simulink model "Simulation"  (R2024a)
settings: Solver=FixedStepAuto  StartTime=0.0  StopTime=0.5  FixedStep=0.1  RelTol=1e-3  EnableMultiTasking=on
settings Model: Creator=hp  LastModifiedBy=Dell

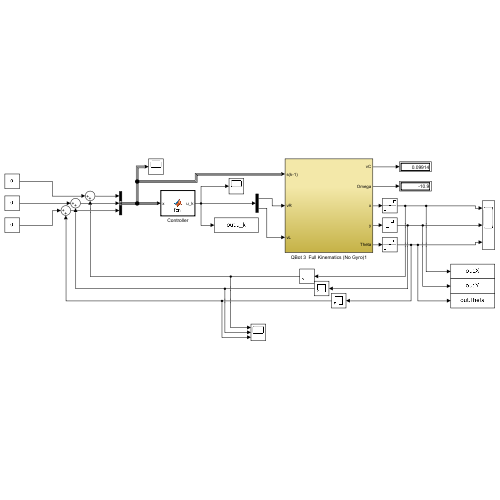
[thumbnail: Simulink's stored preview of the top-level diagram]
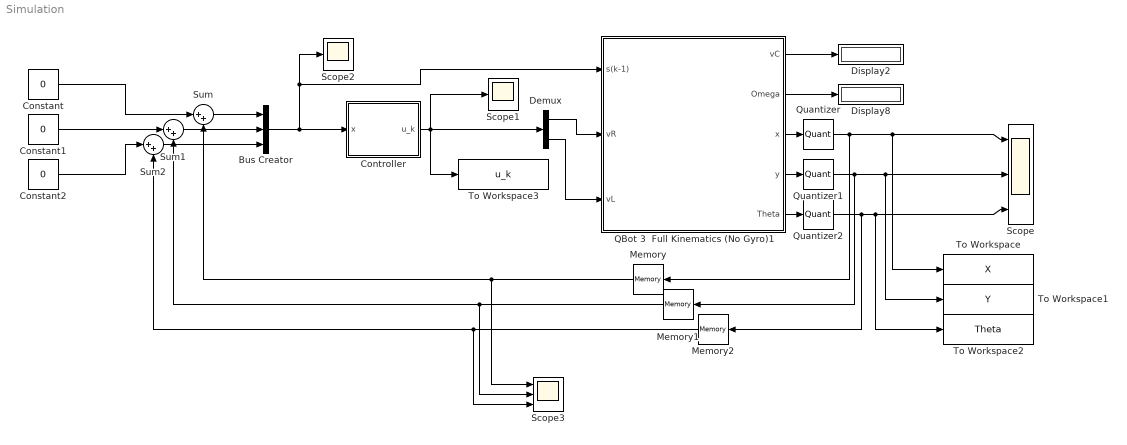
== system Simulation ==
  Bus Creator : BusCreator  Inputs=3
  Constant : Constant  Value=0
  Constant1 : Constant  Value=0
  Constant2 : Constant  Value=0
  Controller : MATLAB Function  TreatAsAtomicUnit=on
  Demux : Demux  Outputs=2
  Display2 : Display
  Display8 : Display
  Memory : Memory  InitialCondition=5
  Memory1 : Memory  InitialCondition=5
  Memory2 : Memory  InitialCondition=9
  QBot 3  Full Kinematics (No Gyro)1 : Subsystem
  Quantizer : Quantizer  QuantizationInterval=-1
  Quantizer1 : Quantizer  QuantizationInterval=-1
  Quantizer2 : Quantizer  QuantizationInterval=-1
  Scope : Scope  NumInputPorts=3
  Scope1 : Scope
  Scope2 : Scope
  Scope3 : Scope  NumInputPorts=3
  Sum : Sum  Inputs=|++
  Sum1 : Sum  Inputs=|++
  Sum2 : Sum  Inputs=|++
  To Workspace : ToWorkspace  VariableName=X  SaveFormat=Timeseries  SampleTime=-1
  To Workspace1 : ToWorkspace  VariableName=Y  SaveFormat=Timeseries  SampleTime=-1
  To Workspace2 : ToWorkspace  VariableName=Theta  SaveFormat=Timeseries  SampleTime=-1
  To Workspace3 : ToWorkspace  VariableName=u_k  SaveFormat=Timeseries  SampleTime=-1
  wires:
  QBot 3  Full Kinematics (No Gyro)1/2(Omega) -> Display8/1
  QBot 3  Full Kinematics (No Gyro)1/1(vC) -> Display2/1
  Demux/1 -> QBot 3  Full Kinematics (No Gyro)1/2(vR)
  Demux/2 -> QBot 3  Full Kinematics (No Gyro)1/3(vL)
  Bus Creator/1 -> QBot 3  Full Kinematics (No Gyro)1/1(s(k-1)), Scope2/1, Controller/1(x)
  Sum/1 -> Bus Creator/1
  Sum1/1 -> Bus Creator/2
  Sum2/1 -> Bus Creator/3
  Memory/1 -> Scope3/1, Sum/2
  Memory1/1 -> Scope3/2, Sum1/2
  Memory2/1 -> Scope3/3, Sum2/2
  Controller/1(u_k) -> Demux/1, Scope1/1, To Workspace3/1
  QBot 3  Full Kinematics (No Gyro)1/3(x) -> Quantizer/1
  QBot 3  Full Kinematics (No Gyro)1/4(y) -> Quantizer1/1
  QBot 3  Full Kinematics (No Gyro)1/5(Theta) -> Quantizer2/1
  Constant/1 -> Sum/1
  Constant1/1 -> Sum1/1
  Constant2/1 -> Sum2/1
  Quantizer/1 -> Memory/1, To Workspace/1, Scope/1
  Quantizer1/1 -> Memory1/1, To Workspace1/1, Scope/2
  Quantizer2/1 -> Memory2/1, To Workspace2/1, Scope/3

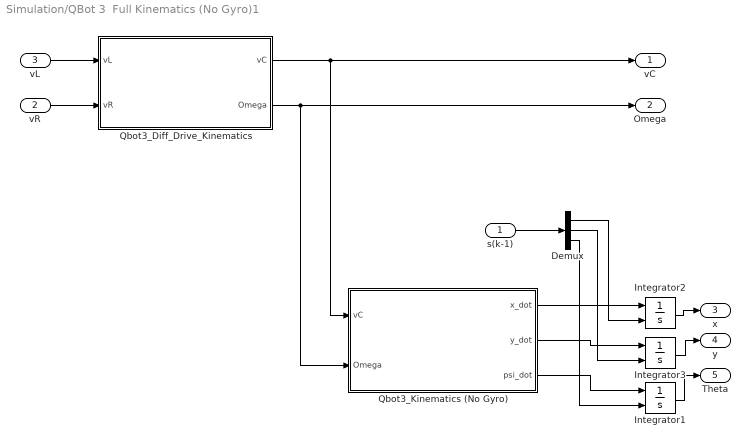
== system Simulation/QBot 3  Full Kinematics (No Gyro)1 ==
  s(k-1) : Inport
  vR : Inport  Port=2
  vL : Inport  Port=3
  Demux : Demux  Outputs=3
  Integrator1 : Integrator  InitialConditionSource=external  InitialCondition=9
  Integrator2 : Integrator  InitialConditionSource=external  InitialCondition=5
  Integrator3 : Integrator  InitialConditionSource=external  InitialCondition=5
  Qbot3_Diff_Drive_Kinematics : Subsystem
  Qbot3_Kinematics (No Gyro) : Subsystem
  vC : Outport
  Omega : Outport  Port=2
  x : Outport  Port=3
  y : Outport  Port=4
  Theta : Outport  Port=5
  wires:
  Qbot3_Kinematics (No Gyro)/2(y_dot) -> Integrator3/1
  Qbot3_Kinematics (No Gyro)/1(x_dot) -> Integrator2/1
  vL/1 -> Qbot3_Diff_Drive_Kinematics/1(vL)
  Qbot3_Diff_Drive_Kinematics/2(Omega) -> Omega/1, Qbot3_Kinematics (No Gyro)/2(Omega)
  Qbot3_Diff_Drive_Kinematics/1(vC) -> vC/1, Qbot3_Kinematics (No Gyro)/1(vC)
  vR/1 -> Qbot3_Diff_Drive_Kinematics/2(vR)
  Qbot3_Kinematics (No Gyro)/3(psi_dot) -> Integrator1/1
  Integrator3/1 -> y/1
  Integrator2/1 -> x/1
  Integrator1/1 -> Theta/1
  s(k-1)/1 -> Demux/1
  Demux/1 -> Integrator2/2
  Demux/2 -> Integrator3/2
  Demux/3 -> Integrator1/2

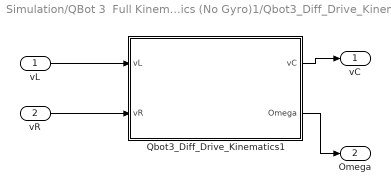
== system Simulation/QBot 3  Full Kinematics (No Gyro)1/Qbot3_Diff_Drive_Kinematics ==
  vL : Inport
  vR : Inport  Port=2
  Qbot3_Diff_Drive_Kinematics1 : MATLAB Function  TreatAsAtomicUnit=on
  vC : Outport
  Omega : Outport  Port=2
  wires:
  vL/1 -> Qbot3_Diff_Drive_Kinematics1/1(vL)
  vR/1 -> Qbot3_Diff_Drive_Kinematics1/2(vR)
  Qbot3_Diff_Drive_Kinematics1/1(vC) -> vC/1
  Qbot3_Diff_Drive_Kinematics1/2(Omega) -> Omega/1

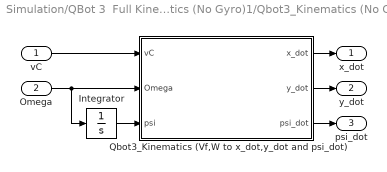
== system Simulation/QBot 3  Full Kinematics (No Gyro)1/Qbot3_Kinematics (No Gyro) ==
  vC : Inport
  Omega : Inport  Port=2
  Integrator : Integrator
  Qbot3_Kinematics (Vf,W to x_dot,y_dot and psi_dot) : MATLAB Function  TreatAsAtomicUnit=on
  x_dot : Outport
  y_dot : Outport  Port=2
  psi_dot : Outport  Port=3
  wires:
  Integrator/1 -> Qbot3_Kinematics (Vf,W to x_dot,y_dot and psi_dot)/3(psi)
  Qbot3_Kinematics (Vf,W to x_dot,y_dot and psi_dot)/1(x_dot) -> x_dot/1
  vC/1 -> Qbot3_Kinematics (Vf,W to x_dot,y_dot and psi_dot)/1(vC)
  Qbot3_Kinematics (Vf,W to x_dot,y_dot and psi_dot)/3(psi_dot) -> psi_dot/1
  Qbot3_Kinematics (Vf,W to x_dot,y_dot and psi_dot)/2(y_dot) -> y_dot/1
  Omega/1 -> Integrator/1, Qbot3_Kinematics (Vf,W to x_dot,y_dot and psi_dot)/2(Omega)

== matlab function Simulation/QBot 3  Full Kinematics (No Gyro)1/Qbot3_Diff_Drive_Kinematics/Qbot3_Diff_Drive_Kinematics1 ==
  data: vL input; vC output; vR input; Omega output
function [vC,Omega] = fcn(vL,vR)

% wheelbase
d= 0.3928;

% calculate forward and turning velocities
vC=0.5*(vL+vR);
Omega=(1/d)*(vR-vL);

== matlab function Simulation/Controller ==
  data: x input; u_k output
function u_k = fcn(x)
    coder.extrinsic('opt_problem');
    H = [1,0,0];
    F = -1.5 ;
    u_k=zeros(1,2);
    gaama = 0.5; %0.5
    c = 0.2; %0.2
    d=0.4;
    dist=0.278; % distance between wheels;
    P0 = eye(3);
    P = eye(3);

    theta=x(3);
    A=eye(3);
    D=0.1.*[0.5*cos(theta), 0.5*cos(theta); 0.5*sin(theta), 0.5*sin(theta);1/dist,-1/dist];
    
    q1 = [2 * x' * A * P * D, -1]';
    q2 = [-H * D, 0]';
    r1 = x' * (A' * P * A - P + c * eye(size(A))) * x;
    r2 = -H * (A + (1 - gaama) * eye(size(A))) * x - (2 - gaama) * F;

    P1=zeros(3,3);
    P1(1:2,1:2) = D' * P * D;
    P2 = 0;

    Uk=opt_problem(P0,P1,P2,q1,q2,r1,r2,d);
    u_k=Uk(1:2);
    d=Uk(3);
end

== matlab function Simulation/QBot 3  Full Kinematics (No Gyro)1/Qbot3_Kinematics (No Gyro)/Qbot3_Kinematics (Vf,W to x_dot,y_dot and psi_dot) ==
  data: vC input; x_dot output; Omega input; y_dot output; psi input; psi_dot output
function [x_dot,y_dot,psi_dot] = fcn(vC,Omega,psi)

% calculate cartesian velocities
x_dot=cos(psi)*vC;
y_dot=sin(psi)*vC;
psi_dot= Omega;
